simulink model "Simscape_motor_model"  (R2019b)
settings: Solver=ode14x  StartTime=0.0  StopTime=0.5  RelTol=1e-3
libraries: fl_lib x6, nesl_utility x5, ee_lib x1
settings Model: Creator=Anas  LastModifiedBy=Anas

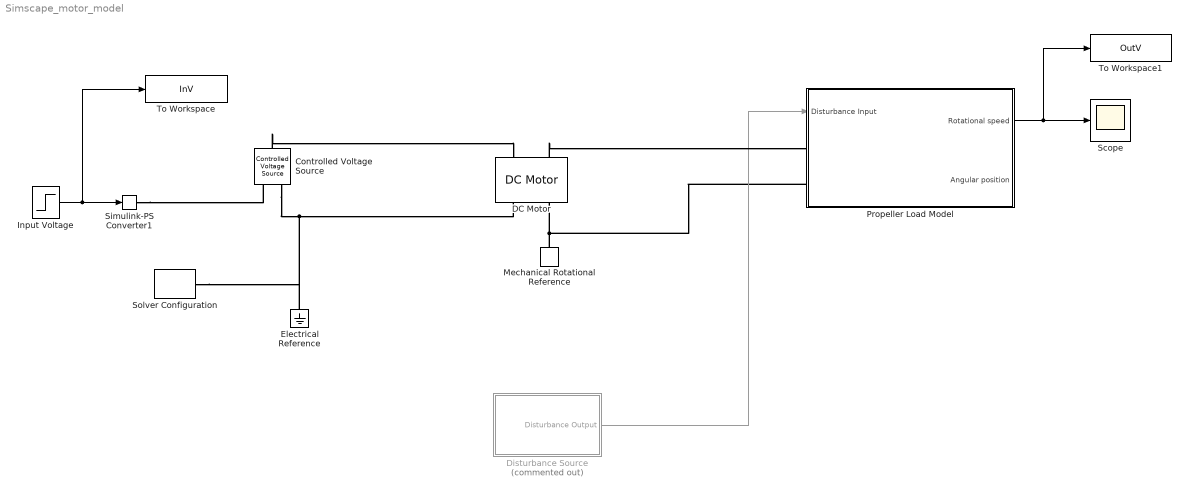
== system Simscape_motor_model ==
  Controlled Voltage Source : fl_lib/Electrical/Electrical Sources/Controlled Voltage Source
  DC Motor : ee_lib/Electromechanical/Brushed Motors/DC Motor  parameterization=3  Ra=3.9 Ohm  La=12e-6 H  emf_or_torque=1  Kv=0.072e-3 V/rpm  Ki=6.876e-4 N*m/A  T_stall=0.24e-3 N*m  w_max=9100 rpm  w_rated=4500 rpm  P_rated=0.462 W  V_rated=6.0 V  J=0.01 g*cm^2  lam_param=2  lam=0 N*m/(rad/s)  i_noload=70 mA  V_i_noload=6.0 V  speed0=0 rpm  alpha=3.93e-3 1/K  Tmeas=25 degC  thermal_mass=100 J/K  initial_temperature=25 degC
      settings: SourceProductName=Simscape Electrical  LogSimulationData=on
  Disturbance Source : Subsystem  Commented=on  VariantControl=Variant1  mask{StepTime=0.2, Tmax=0.0002, Bias=0, Freq=314}
      mask prompts: StepTime "Step Time (s)"; Tmax "Torque (N.m)"; Bias "Bias (N.m)"; Freq "Frequency (rad/s)"
  Electrical Reference : fl_lib/Electrical/Electrical Elements/Electrical Reference
  Input Voltage : Step  Time=0  After=6  SampleTime=0
  Mechanical Rotational Reference : fl_lib/Mechanical/Rotational Elements/Mechanical Rotational Reference
  Propeller Load Model : Subsystem  mask{T=0.00098, J=5e-8, e=0}
      mask prompts: T "Torque (N.m)"; J "Inertia (Kg.m^2)"; e "Coupling Delay"
  Scope : Scope
  Simulink-PS Converter1 : nesl_utility/Simulink-PS Converter  PhysicalDomain=network_engine_domain  SubClassName=ps_input  LeftPortType=input  RightPortType=output  PseudoPeriodic=off  Frequencies=[]  NoiseDistribution=none  NoiseParameters=[]  Unit=1  AffineConversion=off  FilteringAndDerivatives=provide  SimscapeFilterOrder=1  InputFilterTimeConstant=0.001  UdotUserProvided=0
  Solver Configuration : nesl_utility/Solver Configuration  PhysicalDomain=network_engine_domain  SubClassName=solver  LeftPortType=input  RightPortType=generic  Tones=[]  Harmonics=[]  SimulateNoise=off  Profile=off  UseLocalSampling=off  EnableSwitchedLinearOptims=on  FrequencyDomain=off  UseCCode=off  RelTol=0.001  AbsTol=1e-06  MinStep=1e-09  ToWorkspace=off  RevertToSquareIcSolve=off  NumHomotopyIterations=100  PhasorMode=off  PhasorModeNumHarmonics=1  DoDC=off  ResidualTolerance=1e-09  UseLocalSolver=off  LocalSolverChoice=NE_BACKWARD_EULER_ADVANCER  LocalSolverSampleTime=0.001  DoFixedCost=off  MaxNonlinIter=3  MaxModeIter=2  LinearAlgebra=auto  EquationFormulation=NE_TIME_EF  DelaysMemoryBudget=1024  AutomaticFiltering=on  FilteringTimeConstant=0.001  PartitionStorageMethod=AS_NEEDED  PartitionMemoryBudget=1024  PartitionMethod=ROBUST
  To Workspace : ToWorkspace  VariableName=InV  SaveFormat=Timeseries  SampleTime=-1
      settings: Save2DSignal=2-D array (concatenate along first dimension)
  To Workspace1 : ToWorkspace  VariableName=OutV  SaveFormat=Timeseries  SampleTime=-1
  wires:
  Input Voltage/1 -> To Workspace/1, Simulink-PS Converter1/1
  Disturbance Source/1("Disturbance Output ") -> Propeller Load Model/1(Disturbance Input)
  Propeller Load Model/1(Rotational speed) -> To Workspace1/1, Scope/1
  connections:
  Solver Configuration/RConn1 -- Electrical Reference/LConn1 -- Controlled Voltage Source/RConn2 -- DC Motor/RConn1
  Mechanical Rotational Reference/LConn1 -- Propeller Load Model/LConn2 -- DC Motor/RConn2
  Controlled Voltage Source/LConn1 -- DC Motor/LConn1
  Simulink-PS Converter1/RConn1 -- Controlled Voltage Source/RConn1
  DC Motor/LConn2 -- Propeller Load Model/LConn1

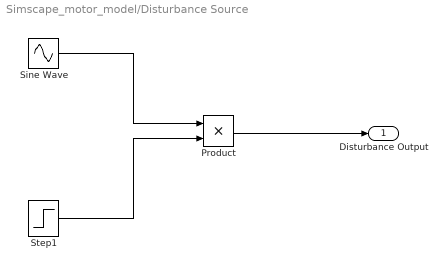
== system Simscape_motor_model/Disturbance Source ==
  Product : Product
  Sine Wave : Sin  Amplitude=Tmax  Bias=Bias  Frequency=Freq  SampleTime=0
  Step1 : Step  Time=StepTime  SampleTime=0
  "Disturbance Output " : Outport
  wires:
  Sine Wave/1 -> Product/1
  Step1/1 -> Product/2
  Product/1 -> "Disturbance Output "/1

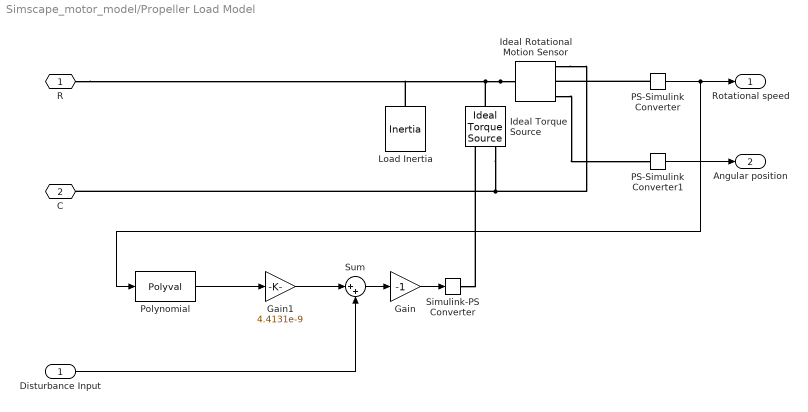
== system Simscape_motor_model/Propeller Load Model ==
  Disturbance Input : Inport
  Gain : Gain  Gain=-1
  Gain1 : Gain  Gain=4.4131e-9
  Ideal Rotational Motion Sensor : fl_lib/Mechanical/Mechanical Sensors/Ideal Rotational Motion Sensor  offset=0 rad
  Ideal Torque Source : fl_lib/Mechanical/Mechanical Sources/Ideal Torque Source
  Load Inertia : fl_lib/Mechanical/Rotational Elements/Inertia  inertia=J kg*m^2  w_specify=off  w_priority=High  w=0 rad/s  w_nominal_specify=off  w_nominal_unit=rad/s  w_nominal_value=1  t_specify=off  t_priority=None  t=0 N*m  t_nominal_specify=off  t_nominal_unit=N*m  t_nominal_value=1
  PS-Simulink Converter : nesl_utility/PS-Simulink Converter  PhysicalDomain=network_engine_domain  SubClassName=ps_output  LeftPortType=input  RightPortType=output  PseudoPeriodic=off  Frequencies=[]  Unit=inherit  AffineConversion=off
  PS-Simulink Converter1 : nesl_utility/PS-Simulink Converter  PhysicalDomain=network_engine_domain  SubClassName=ps_output  LeftPortType=input  RightPortType=output  PseudoPeriodic=off  Frequencies=[]  Unit=inherit  AffineConversion=off
  Polynomial : Polyval  Coefs=[1 0 0 ]
  Simulink-PS Converter : nesl_utility/Simulink-PS Converter  PhysicalDomain=network_engine_domain  SubClassName=ps_input  LeftPortType=input  RightPortType=output  PseudoPeriodic=off  Frequencies=[]  NoiseDistribution=none  NoiseParameters=[]  Unit=1  AffineConversion=off  FilteringAndDerivatives=provide  SimscapeFilterOrder=1  InputFilterTimeConstant=0.001  UdotUserProvided=0
  Sum : Sum  Inputs=|++
  R : PMIOPort  Side=Left
  C : PMIOPort  Port=2  Side=Left
  Rotational speed : Outport
  Angular position : Outport  Port=2
  wires:
  Disturbance Input/1 -> Sum/2
  Gain/1 -> Simulink-PS Converter/1
  Sum/1 -> Gain/1
  Gain1/1 -> Sum/1
  PS-Simulink Converter/1 -> Polynomial/1, Rotational speed/1
  PS-Simulink Converter1/1 -> Angular position/1
  Polynomial/1 -> Gain1/1
  connections:
  Ideal Rotational Motion Sensor/LConn1 -- R/RConn1 -- Load Inertia/LConn1 -- Ideal Torque Source/LConn1
  Ideal Rotational Motion Sensor/RConn1 -- C/RConn1 -- Ideal Torque Source/RConn2
  Simulink-PS Converter/RConn1 -- Ideal Torque Source/RConn1
  PS-Simulink Converter/LConn1 -- Ideal Rotational Motion Sensor/RConn2
  Ideal Rotational Motion Sensor/RConn3 -- PS-Simulink Converter1/LConn1
